simulink model "PT2_model"  (R2015b)
settings: Solver=FixedStepAuto  StartTime=0.0  StopTime=0.2  FixedStep=0.0001  RelTol=1e-3
values from neighbouring files (symbols this model uses):
  CS1 = 1E-6    (= 1e-06)    [parameters.m]
  CS2 = 33E-9    (= 3.3e-08)    [parameters.m]
  RS1 = 20E+3    (= 20000)    [parameters.m]
  RS2 = 20E+3    (= 20000)    [parameters.m]
  Ue = 1    [parameters.m]
libraries: fl_lib x10, nesl_utility x3
settings Model: Creator=lukaskiechle  LastModifiedBy=lukaskiechle

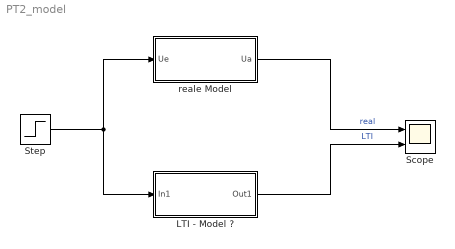
== system PT2_model ==
  LTI - Model ? : Subsystem
  Scope : Scope  NumInputPorts=2
  Step : Step  Time=0.01  After=Ue  SampleTime=0
  reale Model : Subsystem
  wires:
  reale Model/1(Ua) -> Scope/1  "real"
  LTI - Model ?/1(Out1) -> Scope/2  "LTI"
  Step/1 -> LTI - Model ?/1(In1), reale Model/1(Ue)

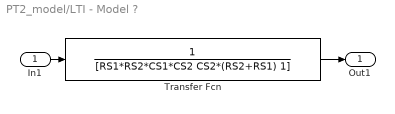
== system PT2_model/LTI - Model ? ==
  In1 : Inport
  Transfer Fcn : TransferFcn  Denominator=[RS1*RS2*CS1*CS2 CS2*(RS2+RS1) 1]
  Out1 : Outport
  wires:
  Transfer Fcn/1 -> Out1/1
  In1/1 -> Transfer Fcn/1

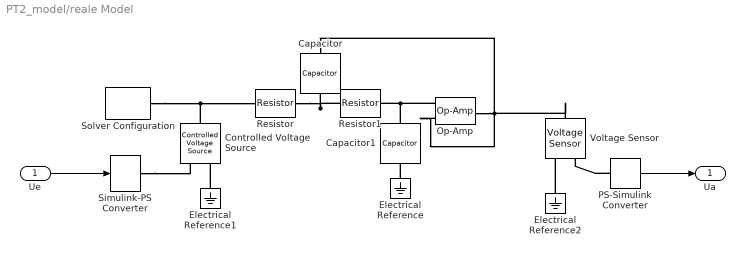
== system PT2_model/reale Model ==
  Ue : Inport
  Capacitor : fl_lib/Electrical/Electrical Elements/Capacitor  c=CS1 F  r=1e-6 Ohm  g=0 1/Ohm  i_specify=off  i_priority=None  i=0 A  v_specify=off  v_priority=None  v=0 V  vc_specify=off  vc_priority=None  vc=0 V
  Capacitor1 : fl_lib/Electrical/Electrical Elements/Capacitor  c=CS2 F  r=1e-6 Ohm  g=0 1/Ohm  i_specify=off  i_priority=None  i=0 A  v_specify=off  v_priority=None  v=0 V  vc_specify=off  vc_priority=None  vc=0 V
  Controlled Voltage Source : fl_lib/Electrical/Electrical Sources/Controlled Voltage Source
  Electrical Reference : fl_lib/Electrical/Electrical Elements/Electrical Reference
  Electrical Reference1 : fl_lib/Electrical/Electrical Elements/Electrical Reference
  Electrical Reference2 : fl_lib/Electrical/Electrical Elements/Electrical Reference
  Op-Amp : fl_lib/Electrical/Electrical Elements/Op-Amp  outI_specify=off  outI_priority=None  outI=0 A
  PS-Simulink Converter : nesl_utility/PS-Simulink Converter  PhysicalDomain=network_engine_domain  SubClassName=ps_output  LeftPortType=input  RightPortType=output  PseudoPeriodic=off  Frequencies=[]  Unit=V  AffineConversion=off
  Resistor : fl_lib/Electrical/Electrical Elements/Resistor  R=RS1 Ohm  i_specify=off  i_priority=None  i=0 A  v_specify=off  v_priority=None  v=0 V
  Resistor1 : fl_lib/Electrical/Electrical Elements/Resistor  R=RS2 Ohm  i_specify=off  i_priority=None  i=0 A  v_specify=off  v_priority=None  v=0 V
  Simulink-PS Converter : nesl_utility/Simulink-PS Converter  PhysicalDomain=network_engine_domain  SubClassName=ps_input  LeftPortType=input  RightPortType=output  PseudoPeriodic=off  Frequencies=[]  NoiseDistribution=none  NoiseParameters=[]  Unit=V  AffineConversion=off  InputFiltering=off  SimscapeFilterOrder=1  InputFilterTimeConstant=0.001  UdotUserProvided=1
  Solver Configuration : nesl_utility/Solver Configuration  PhysicalDomain=network_engine_domain  SubClassName=solver  LeftPortType=input  RightPortType=generic  Accelerate=off  Tones=[]  Harmonics=[]  SimulateNoise=off  Profile=off  UseLocalSampling=off  EnableSwitchedLinearOptims=on  FrequencyDomain=off  UseCCode=off  RelTol=0.001  AbsTol=1e-06  MinStep=1e-09  ToWorkspace=off  RevertToSquareIcSolve=off  NumHomotopyIterations=100  PhasorMode=off  PhasorModeNumHarmonics=1  DoDC=off  ResidualTolerance=1e-09  UseLocalSolver=off  LocalSolverChoice=NE_BACKWARD_EULER_ADVANCER  LocalSolverSampleTime=0.001  DoFixedCost=off  MaxNonlinIter=3  MaxModeIter=2  LinearAlgebra=Sparse  DelaysMemoryBudget=1024  AutomaticFiltering=on  FilteringTimeConstant=0.001
  Voltage Sensor : fl_lib/Electrical/Electrical Sensors/Voltage Sensor
  Ua : Outport
  wires:
  Ue/1 -> Simulink-PS Converter/1
  PS-Simulink Converter/1 -> Ua/1
  connections:
  Op-Amp/LConn2 -- Voltage Sensor/LConn1 -- Capacitor/LConn1 -- Op-Amp/RConn1
  Capacitor/RConn1 -- Resistor/RConn1 -- Resistor1/LConn1
  Capacitor1/LConn1 -- Resistor1/RConn1 -- Op-Amp/LConn1
  Electrical Reference/LConn1 -- Capacitor1/RConn1
  Controlled Voltage Source/LConn1 -- Resistor/LConn1 -- Solver Configuration/RConn1
  Simulink-PS Converter/RConn1 -- Controlled Voltage Source/RConn1
  PS-Simulink Converter/LConn1 -- Voltage Sensor/RConn1
  Electrical Reference1/LConn1 -- Controlled Voltage Source/RConn2
  Electrical Reference2/LConn1 -- Voltage Sensor/RConn2
